simulink model "MotorCntrl"  (R2020b)
settings: Solver=ode45  StartTime=0.0  StopTime=0.4  RelTol=1e-3
values from neighbouring files (symbols this model uses):
  b = 3.5077E-6    [data_dict.sldd]
  J = 3.2284E-6    [data_dict.sldd]
  L = 2.75E-6    [data_dict.sldd]
  R = 4.0    [data_dict.sldd]
undefined symbols (not defined in the file or in its folder): Ke, Kt
settings Model: DataDictionary=motor_dd.sldd  Creator=Sourav Kumar  LastModifiedBy=mluser

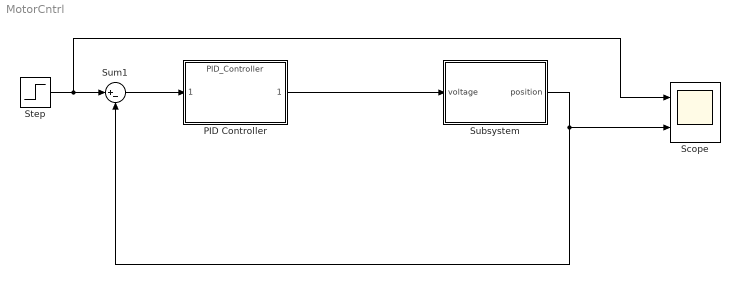
== system MotorCntrl ==
  PID Controller : ModelReference  ModelNameDialog=PID_Controller  SimulationMode=Normal  ModelReferenceVersion=1.5
  Scope : Scope  NumInputPorts=2
  Step : Step  Time=0  SampleTime=0
  Subsystem : Subsystem
  Sum1 : Sum  Inputs=|+-
  wires:
  Step/1 -> Scope/1, Sum1/1
  Sum1/1 -> PID Controller/1
  PID Controller/1 -> Subsystem/1(voltage)
  Subsystem/1(position) -> Scope/2, Sum1/2

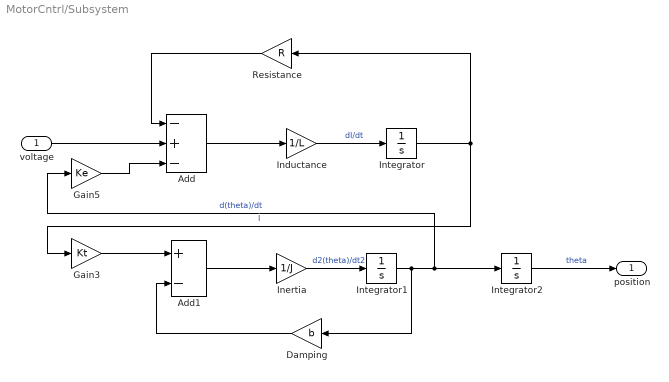
== system MotorCntrl/Subsystem ==
  voltage : Inport
  Add : Sum  Inputs=-+-
  Add1 : Sum  Inputs=+-
  Damping : Gain  Gain=b
  Gain3 : Gain  Gain=Kt
  Gain5 : Gain  Gain=Ke
  Inductance : Gain  Gain=1/L
  Inertia : Gain  Gain=1/J
  Integrator : Integrator
  Integrator1 : Integrator
  Integrator2 : Integrator
  Resistance : Gain  Gain=R
  position : Outport
  wires:
  Integrator1/1 -> Damping/1, Gain5/1, Integrator2/1  "d(theta)/dt"
  Add/1 -> Inductance/1
  Inductance/1 -> Integrator/1  "dI/dt"
  Integrator/1 -> Gain3/1, Resistance/1  "I"
  Resistance/1 -> Add/1
  voltage/1 -> Add/2
  Add1/1 -> Inertia/1
  Integrator2/1 -> position/1  "theta"
  Damping/1 -> Add1/2
  Gain5/1 -> Add/3
  Inertia/1 -> Integrator1/1  "d2(theta)/dt2"
  Gain3/1 -> Add1/1
